simulink model "ball_and_func_2020b"  (R2020b)
settings: Solver=FixedStepAuto  StartTime=0.0  StopTime=100  FixedStep=0.05  RelTol=1e-3
values from neighbouring files (symbols this model uses):
  angle_input_alt = -0.2    [fuzzy_angle_controller.m]
  angle_input_ust = 0.2    [fuzzy_angle_controller.m]
  angular_velocity_alt = -0.6    [fuzzy_angle_controller.m]
  angular_velocity_ust = 0.6    [fuzzy_angle_controller.m]
  angularvelocity_alt = -0.03    [fuzzy_angle_controller.m]
  angularvelocity_ust = 0.03    [fuzzy_angle_controller.m]
  gain1 = 6.270    (= 6.27)    [fuzzy_angle_controller.m]
  gain2 = 5.82    [fuzzy_angle_controller.m]
  gain3 = 15.78    [fuzzy_angle_controller.m]
  gain4 = 1.39    [fuzzy_angle_controller.m]
  input_power_alt = -3    [fuzzy_angle_controller.m]
  input_power_ust = 3    [fuzzy_angle_controller.m]
  position_alt = -0.7    [fuzzy_angle_controller.m]
  position_ust = 0.7    [fuzzy_angle_controller.m]
  speed_alt = -0.5    [fuzzy_angle_controller.m]
  speed_ust = 0.5    [fuzzy_angle_controller.m]
libraries: fuzblock x9
settings Model: Creator=eymen  LastModifiedBy=Mali
settings DataIOCC: ReturnWorkspaceOutputs=off
settings DebuggingCC: SFMachineParentedDataDiag=error

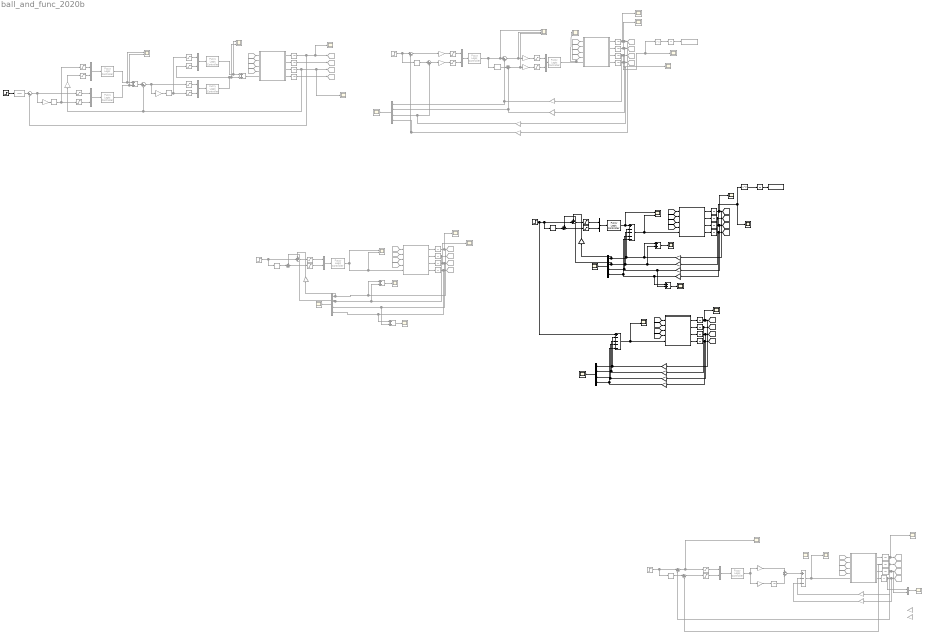
== system ball_and_func_2020b ==
  Add : Sum  Inputs=+----
  Add{1..2,8..9} (4 alike) : Sum  Commented=on
  Add3 : Sum  Commented=on  Inputs=+--
  Add4 : Sum  Inputs=+----
  Add5 : Sum
  Add6 : Sum
  Angle : Saturate  Commented=on  UpperLimit=angle_input_ust  LowerLimit=angle_input_alt
  Angle Controller : fuzblock/Fuzzy Logic  Controller  Commented=on  FIS=angle_fuzzy  OutputSampleNumber=101  DataType=double  FuzzifiedInputs=off  RuleFiringStrengths=off  RuleOutputs=off  AggregatedOutputs=off  SimulateUsing=Interpreted execution  OutOfRangeInputValueMessage=warning  NoRuleFiredMessage=warning  EmptyOutputFuzzySetMessage=warning
  Angle Offset : Saturate  Commented=on  UpperLimit=0.1  LowerLimit=-0.1
  Angular Velocity : Saturate  Commented=on  UpperLimit=angular_velocity_ust  LowerLimit=angular_velocity_alt
  Angular Velocity Saturation : Saturate  Commented=on  UpperLimit=angularvelocity_ust  LowerLimit=angularvelocity_alt
  Ball Friction Observer : fuzblock/Fuzzy Logic  Controller  Commented=on  FIS=ball_friction  OutputSampleNumber=101  DataType=double  FuzzifiedInputs=off  RuleFiringStrengths=off  RuleOutputs=off  AggregatedOutputs=off  SimulateUsing=Interpreted execution  OutOfRangeInputValueMessage=warning  NoRuleFiredMessage=warning  EmptyOutputFuzzySetMessage=warning
  Ball and Beam System : MATLAB Function  TreatAsAtomicUnit=on
  Ball and Beam System1 : MATLAB Function  Commented=on  TreatAsAtomicUnit=on
  Ball and Beam System2 : MATLAB Function  Commented=on  TreatAsAtomicUnit=on
  Ball and Beam System3 : MATLAB Function  Commented=on  TreatAsAtomicUnit=on
  Ball and Beam System4 : MATLAB Function  TreatAsAtomicUnit=on
  Ball and Beam System5 : MATLAB Function  Commented=on  TreatAsAtomicUnit=on
  Beam Friction Observer : fuzblock/Fuzzy Logic  Controller  Commented=on  FIS=beam_friction  OutputSampleNumber=101  DataType=double  FuzzifiedInputs=off  RuleFiringStrengths=off  RuleOutputs=off  AggregatedOutputs=off  SimulateUsing=Interpreted execution  OutOfRangeInputValueMessage=warning  NoRuleFiredMessage=warning  EmptyOutputFuzzySetMessage=warning
  Derivative{,1..2,4..6} (6 alike) : Derivative  Commented=on
  Derivative3 : Derivative
  From{6,10,14,22} (4 alike) : From  Commented=on  GotoTag=x2
  From{7,11,15,23} (4 alike) : From  Commented=on  GotoTag=x3
  From{8,12,16,24} (4 alike) : From  Commented=on  GotoTag=x4
  From{5,9,13,21} (4 alike) : From  Commented=on  GotoTag=x1
  Fuzzy Logic Controller : fuzblock/Fuzzy Logic  Controller  Commented=on  FIS=fuzzy_bb  OutputSampleNumber=101  DataType=double  FuzzifiedInputs=off  RuleFiringStrengths=off  RuleOutputs=off  AggregatedOutputs=off  SimulateUsing=Interpreted execution  OutOfRangeInputValueMessage=warning  NoRuleFiredMessage=warning  EmptyOutputFuzzySetMessage=warning
  Fuzzy Logic Controller1 : fuzblock/Fuzzy Logic  Controller  FIS=position_fuzzy  OutputSampleNumber=101  DataType=double  FuzzifiedInputs=off  RuleFiringStrengths=off  RuleOutputs=off  AggregatedOutputs=off  SimulateUsing=Interpreted execution  OutOfRangeInputValueMessage=warning  NoRuleFiredMessage=warning  EmptyOutputFuzzySetMessage=warning
  Fuzzy Logic Controller2 : fuzblock/Fuzzy Logic  Controller  Commented=on  FIS=angle_fuzzy  OutputSampleNumber=101  DataType=double  FuzzifiedInputs=off  RuleFiringStrengths=off  RuleOutputs=off  AggregatedOutputs=off  SimulateUsing=Interpreted execution  OutOfRangeInputValueMessage=warning  NoRuleFiredMessage=warning  EmptyOutputFuzzySetMessage=warning
  Fuzzy Logic Controller3 : fuzblock/Fuzzy Logic  Controller  Commented=on  FIS=position_fuzzy  OutputSampleNumber=101  DataType=double  FuzzifiedInputs=off  RuleFiringStrengths=off  RuleOutputs=off  AggregatedOutputs=off  SimulateUsing=Interpreted execution  OutOfRangeInputValueMessage=warning  NoRuleFiredMessage=warning  EmptyOutputFuzzySetMessage=warning
  Fuzzy Logic Controller4 : fuzblock/Fuzzy Logic  Controller  Commented=on  FIS=position_fuzzy  OutputSampleNumber=101  DataType=double  FuzzifiedInputs=off  RuleFiringStrengths=off  RuleOutputs=off  AggregatedOutputs=off  SimulateUsing=Interpreted execution  OutOfRangeInputValueMessage=warning  NoRuleFiredMessage=warning  EmptyOutputFuzzySetMessage=warning
  Gain : Gain  Gain=gain1
  Gain1 : Gain  Gain=gain2
  Gain10 : Gain  Gain=8
  Gain11 : Gain  Gain=gain1
  Gain12 : Gain  Commented=on  Gain=-1
  Gain13 : Gain  Commented=on  Gain=-1
  Gain14 : Gain  Commented=on  Gain=-1
  Gain15 : Gain  Gain=gain2
  Gain16 : Gain  Gain=gain3
  Gain17 : Gain  Gain=gain4
  Gain{18..21} (4 alike) : Gain  Commented=on
  Gain2 : Gain  Gain=gain3
  Gain22 : Gain  Commented=on  Gain=gain3
  Gain23 : Gain  Commented=on  Gain=gain4
  Gain24 : Gain  Commented=on  Gain=gain1
  Gain25 : Gain  Commented=on  Gain=gain2
  Gain28 : Gain  Commented=on  Gain=8
  Gain3 : Gain  Gain=gain4
  Gain4 : Gain  Commented=on  Gain=12
  Gain5 : Gain  Commented=on  Gain=18
  Gain6 : Gain  Commented=on  Gain=58.78
  Gain7 : Gain  Commented=on  Gain=6.39
  Gain8 : Gain  Commented=on  Gain=27.170
  Gain9 : Gain  Commented=on  Gain=29.82
  Goto{6,10,14,22} (4 alike) : Goto  Commented=on  GotoTag=x2
  Goto{7,11,15,23} (4 alike) : Goto  Commented=on  GotoTag=x3
  Goto{8,12,16,24} (4 alike) : Goto  Commented=on  GotoTag=x4
  Goto{5,9,13,21} (4 alike) : Goto  Commented=on  GotoTag=x1
  Integrator{,1..3,13,18..20,22} (9 alike) : Integrator
  Integrator{4..12,14..17,21,23..25,27} (18 alike) : Integrator  Commented=on
  Mux : Mux  Inputs=2
  Mux{1..5,7..8,10,12} (9 alike) : Mux  Commented=on  Inputs=2
  Mux11 : Mux  Commented=on
  Mux13 : Mux  Commented=on
  Mux6 : Mux
  Mux9 : Mux
  Position Controller : fuzblock/Fuzzy Logic  Controller  Commented=on  FIS=position_fuzzy  OutputSampleNumber=101  DataType=double  FuzzifiedInputs=off  RuleFiringStrengths=off  RuleOutputs=off  AggregatedOutputs=off  SimulateUsing=Interpreted execution  OutOfRangeInputValueMessage=warning  NoRuleFiredMessage=warning  EmptyOutputFuzzySetMessage=warning
  Position Saturation : Saturate  Commented=on  UpperLimit=position_ust  LowerLimit=position_alt
  Power Offset Saturation : Saturate  Commented=on  UpperLimit=input_power_ust  LowerLimit=input_power_alt
  Saturation : Saturate  Commented=on  UpperLimit=position_ust  LowerLimit=position_alt
  Saturation1 : Saturate  Commented=on  UpperLimit=speed_ust  LowerLimit=speed_alt
  Saturation2 : Saturate  UpperLimit=position_ust  LowerLimit=position_alt
  Saturation3 : Saturate  UpperLimit=speed_ust  LowerLimit=speed_alt
  Saturation4 : Saturate  Commented=on  UpperLimit=angle_input_ust  LowerLimit=angle_input_alt
  Saturation5 : Saturate  Commented=on  UpperLimit=angular_velocity_ust  LowerLimit=angular_velocity_alt
  Saturation6 : Saturate  Commented=on  UpperLimit=position_ust  LowerLimit=position_alt
  Saturation7 : Saturate  Commented=on  UpperLimit=speed_ust  LowerLimit=speed_alt
  Saturation8 : Saturate  Commented=on  UpperLimit=position_ust  LowerLimit=position_alt
  Saturation9 : Saturate  Commented=on  UpperLimit=speed_ust  LowerLimit=speed_alt
  Scope : Scope  NumInputPorts=2
  Scope{1..2,5..10,13..14,21..23,26..30} (18 alike) : Scope  Commented=on
  Scope11 : Scope  NumInputPorts=2
  Scope{12,15..19,24} (7 alike) : Scope
  Scope20 : Scope  Commented=on  NumInputPorts=3
  Scope25 : Scope  Commented=on  NumInputPorts=2
  Scope3 : Scope  Commented=on  NumInputPorts=2
  Scope4 : Scope  Commented=on  NumInputPorts=2
  Speed Saturation : Saturate  Commented=on  UpperLimit=0.1  LowerLimit=-0.1
  Speed_Saturation : Saturate  Commented=on  UpperLimit=speed_ust  LowerLimit=speed_alt
  Square : Math  Commented=on  Operator=square  SaturateOnIntegerOverflow=on
  Square1 : Math  Operator=square  SaturateOnIntegerOverflow=on
  Step : Step  SampleTime=0
  Step1 : Step  Commented=on  SampleTime=0
  Step2 : Step  SampleTime=0
  Step3 : Step  Commented=on  SampleTime=0
  Step4 : Step  Commented=on  SampleTime=0
  Sum{,1..3} (4 alike) : Sum  Commented=on  Inputs=|+-
  Sum{7..10} (4 alike) : Sum  Commented=on  Inputs=|++
  Sum11 : Sum  Commented=on  Inputs=++|
  Sum12 : Sum  Commented=on  Inputs=++|
  Sum4 : Sum  Commented=on  Inputs=+|+
  Sum5 : Sum  Inputs=++|
  Sum6 : Sum  Inputs=++|
  To Workspace : ToWorkspace  Commented=on  VariableName=ISE  SampleTime=-1
      settings: Save2DSignal=2-D array (concatenate along first dimension)
  To Workspace2 : ToWorkspace  VariableName=ise  SampleTime=-1
      settings: Save2DSignal=2-D array (concatenate along first dimension)
  Transfer Fcn : TransferFcn  Commented=on  Denominator=[1 1]
  wires:
  Ball and Beam System/1(d_x1) -> Integrator/1
  Ball and Beam System/2(d_x2) -> Integrator1/1
  Ball and Beam System/3(d_x3) -> Integrator2/1
  Ball and Beam System/4(d_x4) -> Integrator3/1
  Integrator1/1 -> [x2], Gain1/1
  Integrator/1 -> Scope17/1, Gain/1, [x1]  "ball position"
  [x4] -> Ball and Beam System/4(x4)
  [x3] -> Ball and Beam System/3(x3)
  [x2] -> Ball and Beam System/2(x2)
  [x1] -> Ball and Beam System/1(x1)
  Add/1 -> Scope/2, Ball and Beam System/5(u)
  Integrator3/1 -> [x4], Gain3/1
  Gain/1 -> Add5/1, Add/2, Mux6/1, Gain10/1  "ball_position"
  Gain1/1 -> Add5/2, Sum6/1, Mux6/2, Add/3  "velocity of the ball"
  Gain2/1 -> Add6/2, Add/4, Mux6/3  "angle of the beam"
  Gain3/1 -> Add6/1, Add/5, Mux6/4  "angular velocity of the beam"
  Integrator6/1 -> Scope2/1, Goto7/1, Gain12/1, Sum/2  "angle"
  From5/1 -> Ball and Beam System1/1(x1)
  From6/1 -> Ball and Beam System1/2(x2)
  Ball and Beam System1/2(d_x2) -> Integrator5/1
  Ball and Beam System1/1(d_x1) -> Integrator4/1
  From8/1 -> Ball and Beam System1/4(x4)
  Ball and Beam System1/4(d_x4) -> Integrator7/1
  Ball and Beam System1/3(d_x3) -> Integrator6/1
  From7/1 -> Ball and Beam System1/3(x3)
  Integrator7/1 -> Goto8/1
  Integrator4/1 -> Sum1/2, Scope5/1, Goto5/1
  Integrator5/1 -> Goto6/1
  Add1/1 -> Ball and Beam System1/5(u)
  Angle Controller/1 -> Power Offset Saturation/1, Add1/2, Scope3/2
  Beam Friction Observer/1 -> Scope3/1, Add1/1
  Mux1/1 -> Beam Friction Observer/1
  Angular Velocity Saturation/1 -> Mux1/1
  Power Offset Saturation/1 -> Mux1/2
  Angle/1 -> Mux2/1
  Angular Velocity/1 -> Mux2/2
  Mux2/1 -> Angle Controller/1
  Sum/1 -> Angle/1, Gain14/1
  Derivative/1 -> Angular Velocity Saturation/1, Angular Velocity/1
  Add2/1 -> Sum/1
  Position Controller/1 -> Scope4/2, Add2/2
  Ball Friction Observer/1 -> Scope4/1, Add2/1
  Mux3/1 -> Position Controller/1
  Mux4/1 -> Ball Friction Observer/1
  Speed Saturation/1 -> Mux4/1
  Angle Offset/1 -> Mux4/2
  Position Saturation/1 -> Mux3/1
  Speed_Saturation/1 -> Mux3/2
  Sum1/1 -> Gain13/1, Position Saturation/1
  Derivative1/1 -> Speed Saturation/1, Speed_Saturation/1
  Transfer Fcn/1 -> Sum1/1
  Step/1 -> Transfer Fcn/1
  Mux5/1 -> Scope6/1
  Gain7/1 -> Add3/3
  Gain6/1 -> Add3/2
  Integrator11/1 -> Mux5/1, Goto12/1, Gain7/1
  Add3/1 -> Scope8/1, Ball and Beam System2/5(u)
  From9/1 -> Ball and Beam System2/1(x1)
  From10/1 -> Ball and Beam System2/2(x2)
  From11/1 -> Ball and Beam System2/3(x3)
  From12/1 -> Ball and Beam System2/4(x4)
  Integrator10/1 -> Goto11/1, Mux5/2, Gain6/1  "angle"
  Ball and Beam System2/4(d_x4) -> Integrator11/1
  Ball and Beam System2/3(d_x3) -> Integrator10/1
  Ball and Beam System2/2(d_x2) -> Integrator9/1
  Ball and Beam System2/1(d_x1) -> Integrator8/1
  Step1/1 -> Derivative2/1, Sum2/1  "ref"
  Mux7/1 -> Fuzzy Logic Controller/1
  Saturation/1 -> Mux7/1
  Saturation1/1 -> Mux7/2
  Derivative2/1 -> Sum3/1
  Sum2/1 -> Saturation/1, Scope9/1
  Sum3/1 -> Saturation1/1
  Integrator9/1 -> Sum3/2, Goto10/1
  Integrator8/1 -> Sum2/2, Goto9/1, Scope7/1
  Sum4/1 -> Add3/1
  Integrator12/1 -> Sum4/2
  Gain4/1 -> Integrator12/1
  Fuzzy Logic Controller/1 -> Gain4/1, Gain5/1
  Gain5/1 -> Sum4/1
  Mux/1 -> Fuzzy Logic Controller1/1
  Saturation3/1 -> Mux/2
  Derivative3/1 -> Sum6/2
  Sum6/1 -> Saturation3/1
  Sum5/1 -> Saturation2/1
  Saturation2/1 -> Mux/1
  Step2/1 -> Add4/1, Derivative3/1, Sum5/2
  Fuzzy Logic Controller1/1 -> Scope/1, Add/1
  Mux6/1 -> Scope12/1
  Integrator17/1 -> Scope22/1, Gain23/1, Goto16/1  "beam velo"
  From13/1 -> Ball and Beam System3/1(x1)
  From14/1 -> Ball and Beam System3/2(x2)
  From15/1 -> Ball and Beam System3/3(x3)
  From16/1 -> Ball and Beam System3/4(x4)
  Integrator14/1 -> Scope1/1, Gain24/1, Goto13/1  "ball position"
  Integrator16/1 -> Square/1, Scope13/1, Goto15/1, Gain22/1  "beam angle"
  Integrator15/1 -> Scope23/1, Gain25/1, Goto14/1  "ball velocity"
  Ball and Beam System3/4(d_x4) -> Integrator17/1
  Ball and Beam System3/3(d_x3) -> Integrator16/1
  Ball and Beam System3/2(d_x2) -> Integrator15/1
  Ball and Beam System3/1(d_x1) -> Integrator14/1
  Gain12/1 -> Angle Offset/1
  Gain13/1 -> Derivative1/1
  Gain14/1 -> Derivative/1
  Gain10/1 -> Sum5/1
  Gain17/1 -> Mux9/4, Add4/5  "angular velocity of the beam"
  Gain16/1 -> Mux9/3, Add4/4  "agle of the beam"
  Gain15/1 -> Mux9/2, Add4/3  "velocity of the ball"
  Gain11/1 -> Mux9/1, Add4/2  "ball_position"
  Integrator20/1 -> Gain17/1, [x4_]
  Add4/1 -> Ball and Beam System4/5(u), Scope11/2
  [x1_] -> Ball and Beam System4/1(x1)
  [x2_] -> Ball and Beam System4/2(x2)
  [x3_] -> Ball and Beam System4/3(x3)
  [x4_] -> Ball and Beam System4/4(x4)
  Integrator13/1 -> Scope16/1, [x1_], Gain11/1  "ball position"
  Integrator19/1 -> [x3_], Gain16/1  "angle"
  Integrator18/1 -> Gain15/1, [x2_]
  Ball and Beam System4/4(d_x4) -> Integrator20/1
  Ball and Beam System4/3(d_x3) -> Integrator19/1
  Ball and Beam System4/2(d_x2) -> Integrator18/1
  Ball and Beam System4/1(d_x1) -> Integrator13/1
  Mux9/1 -> Scope15/1
  Add5/1 -> Scope18/1
  Add6/1 -> Scope19/1
  Mux8/1 -> Fuzzy Logic Controller2/1
  Saturation4/1 -> Mux8/1
  Saturation5/1 -> Mux8/2
  Gain18/1 -> Saturation4/1
  Gain19/1 -> Saturation5/1
  Sum7/1 -> Scope20/2, Gain18/1
  Fuzzy Logic Controller3/1 -> Derivative4/1, Scope20/1, Sum7/1
  Sum9/1 -> Scope20/3, Gain19/1
  Square/1 -> Integrator21/1
  Integrator21/1 -> To Workspace/1
  Saturation7/1 -> Mux10/2
  Gain20/1 -> Saturation6/1
  Gain21/1 -> Saturation7/1
  Mux10/1 -> Fuzzy Logic Controller3/1
  Step3/1 -> Derivative5/1, Sum8/1
  Sum10/1 -> Gain21/1
  Sum8/1 -> Gain20/1
  Saturation6/1 -> Mux10/1
  Gain22/1 -> Mux11/1, Sum7/2  "beam angle"
  Fuzzy Logic Controller2/1 -> Scope14/1, Ball and Beam System3/5(u)
  Gain23/1 -> Mux11/2, Sum9/2  "beam velo"
  Gain24/1 -> Mux11/4, Sum8/2  "ball pos"
  Gain25/1 -> Mux11/3, Sum10/2  "ball velo"
  Mux11/1 -> Scope21/1
  Derivative5/1 -> Sum10/1
  Derivative4/1 -> Sum9/1
  Square1/1 -> Integrator22/1
  Integrator2/1 -> Scope24/1, Square1/1, Gain2/1, [x3]  "beam angle"
  Integrator22/1 -> To Workspace2/1
  Ball and Beam System5/4(d_x4) -> Integrator27/1
  Integrator23/1 -> Add8/1, Mux13/1, Gain28/1, Scope27/1, Goto21/1  "ball_position"
  Integrator27/1 -> Add9/1, Mux13/4, Goto24/1  "angular velocity of the beam"
  Ball and Beam System5/2(d_x2) -> Integrator24/1
  Integrator25/1 -> Scope30/1, Add9/2, Mux13/3, Goto23/1  "beam angle"
  From24/1 -> Ball and Beam System5/4(x4)
  From22/1 -> Ball and Beam System5/2(x2)
  From21/1 -> Ball and Beam System5/1(x1)
  Ball and Beam System5/1(d_x1) -> Integrator23/1
  Step4/1 -> Derivative6/1, Sum11/2
  Sum12/1 -> Saturation9/1
  Mux12/1 -> Fuzzy Logic Controller4/1
  Sum11/1 -> Saturation8/1
  Derivative6/1 -> Sum12/2
  From23/1 -> Ball and Beam System5/3(x3)
  Mux13/1 -> Scope26/1
  Saturation9/1 -> Mux12/2
  Gain28/1 -> Sum11/1
  Integrator24/1 -> Add8/2, Sum12/1, Mux13/2, Goto22/1  "velocity of the ball"
  Add8/1 -> Scope28/1
  Saturation8/1 -> Mux12/1
  Add9/1 -> Scope29/1
  Ball and Beam System5/3(d_x3) -> Integrator25/1
  Fuzzy Logic Controller4/1 -> Ball and Beam System5/5(u), Scope25/2, Scope25/1

== matlab function ball_and_func_2020b/Ball and Beam System1 ==
  data: x1 input; x2 input; x3 input; x4 input; u input; d_x1 output; d_x2 output; d_x3 output; d_x4 output
function [d_x1, d_x2, d_x3, d_x4] = fcn(x1, x2, x3, x4, u)

R = 0.02;
m = 0.27;
M = 1.122;
Iw = 0.5;
l = 0.49;
D = 0.017;
b = 1;
K = 0.001;
g = 9.8;

r = sqrt(R^2 -(D/2)^2);
Ib = 0.4*m*R^2;
Ii = (1/3)*Iw^2*M;
Im = 0.5*Ii;
Iw = Ii + Im;

a1 = m + Ib/r^2;
a2 = (m*r^2 + Ib)/r;
a3 = m*g;

b1 = Ib + Iw;
b2 = 2*m;
b3 = b*l^2;
b4 = K*l^2;
b5 = (m*r^2 + Ib)/r;
b6 = m*g;

d_x1 = x2;

d_x2 = (a2*((b2*x1*x2 + b3)*x4 + b4*x3 - b6*x1*cos(x3))+ (m*x1^2 + b1)*(a3*sin(x3)+m*x1*x4^2)-a2*l*cos(x3)*u)/(a1*(m*x1^2+b1)-a2*b5);

d_x3 = x4;

d_x4 = (-(b2*x1*x2 + b3)*x4 - b4*x3 + b6*x1*cos(x3))/(m*x1^2 + b1)-(b5*(a3*sin(x3)+m*x1*x4^2))/(a1*(m*x1^2 + b1)-a2*b5)-(a2*b5*((b2*x1*x2+b3)*x4 + b4*x3 - b6*x1*cos(x3)))/((m*x1^2+b1)*(a1*(m*x1^2+b1)-a2*b5))+(1+(a2*b5)/(a1*(m*x1^2+b1)-a2*b5))*((l*cos(x3)*u)/(m*x1^2+b1));

== matlab function ball_and_func_2020b/Ball and Beam System ==
  data: x1 input; x2 input; x3 input; x4 input; u input; d_x1 output; d_x2 output; d_x3 output; d_x4 output
function [d_x1, d_x2, d_x3, d_x4] = fcn(x1, x2, x3, x4, u)

R = 0.02;
m = 0.27;
M = 1.122;
Iw = 0.5;
l = 0.49;
D = 0.017;
b = 1;
K = 0.001;
g = 9.8;

r = sqrt(R^2 -(D/2)^2);
Ib = 0.4*m*R^2;
Ii = (1/3)*Iw^2*M;
Im = 0.5*Ii;
Iw = Ii + Im;

a1 = m + Ib/r^2;
a2 = (m*r^2 + Ib)/r;
a3 = m*g;

b1 = Ib + Iw;
b2 = 2*m;
b3 = b*l^2;
b4 = K*l^2;
b5 = (m*r^2 + Ib)/r;
b6 = m*g;

d_x1 = x2;

d_x2 = (a2*((b2*x1*x2 + b3)*x4 + b4*x3 - b6*x1*cos(x3))+ (m*x1^2 + b1)*(a3*sin(x3)+m*x1*x4^2)-a2*l*cos(x3)*u)/(a1*(m*x1^2+b1)-a2*b5);

d_x3 = x4;

d_x4 = (-(b2*x1*x2 + b3)*x4 - b4*x3 + b6*x1*cos(x3))/(m*x1^2 + b1)-(b5*(a3*sin(x3)+m*x1*x4^2))/(a1*(m*x1^2 + b1)-a2*b5)-(a2*b5*((b2*x1*x2+b3)*x4 + b4*x3 - b6*x1*cos(x3)))/((m*x1^2+b1)*(a1*(m*x1^2+b1)-a2*b5))+(1+(a2*b5)/(a1*(m*x1^2+b1)-a2*b5))*((l*cos(x3)*u)/(m*x1^2+b1));

== matlab function ball_and_func_2020b/Ball and Beam System2 ==
  data: x1 input; x2 input; x3 input; x4 input; u input; d_x1 output; d_x2 output; d_x3 output; d_x4 output
function [d_x1, d_x2, d_x3, d_x4] = fcn(x1, x2, x3, x4, u)

R = 0.02;
m = 0.27;
M = 1.122;
Iw = 0.5;
l = 0.49;
D = 0.017;
b = 1;
K = 0.001;
g = 9.8;

r = sqrt(R^2 -(D/2)^2);
Ib = 0.4*m*R^2;
Ii = (1/3)*Iw^2*M;
Im = 0.5*Ii;
Iw = Ii + Im;

a1 = m + Ib/r^2;
a2 = (m*r^2 + Ib)/r;
a3 = m*g;

b1 = Ib + Iw;
b2 = 2*m;
b3 = b*l^2;
b4 = K*l^2;
b5 = (m*r^2 + Ib)/r;
b6 = m*g;

d_x1 = x2;

d_x2 = (a2*((b2*x1*x2 + b3)*x4 + b4*x3 - b6*x1*cos(x3))+ (m*x1^2 + b1)*(a3*sin(x3)+m*x1*x4^2)-a2*l*cos(x3)*u)/(a1*(m*x1^2+b1)-a2*b5);

d_x3 = x4;

d_x4 = (-(b2*x1*x2 + b3)*x4 - b4*x3 + b6*x1*cos(x3))/(m*x1^2 + b1)-(b5*(a3*sin(x3)+m*x1*x4^2))/(a1*(m*x1^2 + b1)-a2*b5)-(a2*b5*((b2*x1*x2+b3)*x4 + b4*x3 - b6*x1*cos(x3)))/((m*x1^2+b1)*(a1*(m*x1^2+b1)-a2*b5))+(1+(a2*b5)/(a1*(m*x1^2+b1)-a2*b5))*((l*cos(x3)*u)/(m*x1^2+b1));

== matlab function ball_and_func_2020b/Ball and Beam System3 ==
  data: x1 input; x2 input; x3 input; x4 input; u input; d_x1 output; d_x2 output; d_x3 output; d_x4 output
function [d_x1, d_x2, d_x3, d_x4] = fcn(x1, x2, x3, x4, u)

R = 0.02;
m = 0.27;
M = 1.122;
Iw = 0.5;
l = 0.49;
D = 0.017;
b = 1;
K = 0.001;
g = 9.8;

r = sqrt(R^2 -(D/2)^2);
Ib = 0.4*m*R^2;
Ii = (1/3)*Iw^2*M;
Im = 0.5*Ii;
Iw = Ii + Im;

a1 = m + Ib/r^2;
a2 = (m*r^2 + Ib)/r;
a3 = m*g;

b1 = Ib + Iw;
b2 = 2*m;
b3 = b*l^2;
b4 = K*l^2;
b5 = (m*r^2 + Ib)/r;
b6 = m*g;

d_x1 = x2;

d_x2 = (a2*((b2*x1*x2 + b3)*x4 + b4*x3 - b6*x1*cos(x3))+ (m*x1^2 + b1)*(a3*sin(x3)+m*x1*x4^2)-a2*l*cos(x3)*u)/(a1*(m*x1^2+b1)-a2*b5);

d_x3 = x4;

d_x4 = (-(b2*x1*x2 + b3)*x4 - b4*x3 + b6*x1*cos(x3))/(m*x1^2 + b1)-(b5*(a3*sin(x3)+m*x1*x4^2))/(a1*(m*x1^2 + b1)-a2*b5)-(a2*b5*((b2*x1*x2+b3)*x4 + b4*x3 - b6*x1*cos(x3)))/((m*x1^2+b1)*(a1*(m*x1^2+b1)-a2*b5))+(1+(a2*b5)/(a1*(m*x1^2+b1)-a2*b5))*((l*cos(x3)*u)/(m*x1^2+b1));

== matlab function ball_and_func_2020b/Ball and Beam System4 ==
  data: x1 input; x2 input; x3 input; x4 input; u input; d_x1 output; d_x2 output; d_x3 output; d_x4 output
function [d_x1, d_x2, d_x3, d_x4] = fcn(x1, x2, x3, x4, u)

R = 0.02;
m = 0.27;
M = 1.122;
Iw = 0.5;
l = 0.49;
D = 0.017;
b = 1;
K = 0.001;
g = 9.8;

r = sqrt(R^2 -(D/2)^2);
Ib = 0.4*m*R^2;
Ii = (1/3)*Iw^2*M;
Im = 0.5*Ii;
Iw = Ii + Im;

a1 = m + Ib/r^2;
a2 = (m*r^2 + Ib)/r;
a3 = m*g;

b1 = Ib + Iw;
b2 = 2*m;
b3 = b*l^2;
b4 = K*l^2;
b5 = (m*r^2 + Ib)/r;
b6 = m*g;

d_x1 = x2;

d_x2 = (a2*((b2*x1*x2 + b3)*x4 + b4*x3 - b6*x1*cos(x3))+ (m*x1^2 + b1)*(a3*sin(x3)+m*x1*x4^2)-a2*l*cos(x3)*u)/(a1*(m*x1^2+b1)-a2*b5);

d_x3 = x4;

d_x4 = (-(b2*x1*x2 + b3)*x4 - b4*x3 + b6*x1*cos(x3))/(m*x1^2 + b1)-(b5*(a3*sin(x3)+m*x1*x4^2))/(a1*(m*x1^2 + b1)-a2*b5)-(a2*b5*((b2*x1*x2+b3)*x4 + b4*x3 - b6*x1*cos(x3)))/((m*x1^2+b1)*(a1*(m*x1^2+b1)-a2*b5))+(1+(a2*b5)/(a1*(m*x1^2+b1)-a2*b5))*((l*cos(x3)*u)/(m*x1^2+b1));

== matlab function ball_and_func_2020b/Ball and Beam System5 ==
  data: x1 input; x2 input; x3 input; x4 input; u input; d_x1 output; d_x2 output; d_x3 output; d_x4 output
function [d_x1, d_x2, d_x3, d_x4] = fcn(x1, x2, x3, x4, u)

R = 0.02;
m = 0.27;
M = 1.122;
Iw = 0.5;
l = 0.49;
D = 0.017;
b = 1;
K = 0.001;
g = 9.8;

r = sqrt(R^2 -(D/2)^2);
Ib = 0.4*m*R^2;
Ii = (1/3)*Iw^2*M;
Im = 0.5*Ii;
Iw = Ii + Im;

a1 = m + Ib/r^2;
a2 = (m*r^2 + Ib)/r;
a3 = m*g;

b1 = Ib + Iw;
b2 = 2*m;
b3 = b*l^2;
b4 = K*l^2;
b5 = (m*r^2 + Ib)/r;
b6 = m*g;

d_x1 = x2;

d_x2 = (a2*((b2*x1*x2 + b3)*x4 + b4*x3 - b6*x1*cos(x3))+ (m*x1^2 + b1)*(a3*sin(x3)+m*x1*x4^2)-a2*l*cos(x3)*u)/(a1*(m*x1^2+b1)-a2*b5);

d_x3 = x4;

d_x4 = (-(b2*x1*x2 + b3)*x4 - b4*x3 + b6*x1*cos(x3))/(m*x1^2 + b1)-(b5*(a3*sin(x3)+m*x1*x4^2))/(a1*(m*x1^2 + b1)-a2*b5)-(a2*b5*((b2*x1*x2+b3)*x4 + b4*x3 - b6*x1*cos(x3)))/((m*x1^2+b1)*(a1*(m*x1^2+b1)-a2*b5))+(1+(a2*b5)/(a1*(m*x1^2+b1)-a2*b5))*((l*cos(x3)*u)/(m*x1^2+b1));
